simulink model "motorPos_ControlModel"  (R2020a)
settings: Solver=VariableStepAuto  StartTime=0.0  StopTime=10.0  RelTol=1e-3
values from neighbouring files (symbols this model uses):
  Kd = 0.084    [motor_parameter.sldd]
  Ki = 62.72    [motor_parameter.sldd]
  Kp = 4.023    [motor_parameter.sldd]
settings Model: DataDictionary=motor_parameter.sldd  Creator=INDRAJIT MARATHE  LastModifiedBy=INDRAJIT MARATHE

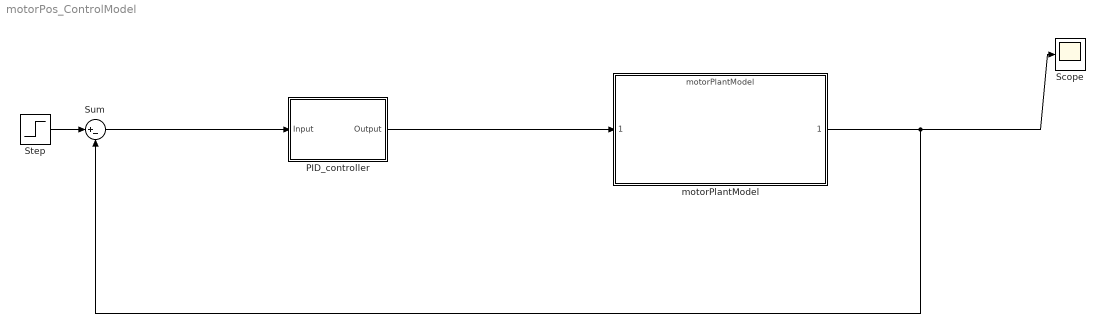
== system motorPos_ControlModel ==
  PID_controller : Subsystem
  Scope : Scope
  Step : Step  SampleTime=0
  Sum : Sum  Inputs=|+-
  motorPlantModel : ModelReference  ModelNameDialog=motorPlantModel  ModelReferenceVersion=1.11
  wires:
  Step/1 -> Sum/1
  motorPlantModel/1 -> Scope/1, Sum/2
  PID_controller/1(Output) -> motorPlantModel/1
  Sum/1 -> PID_controller/1(Input)

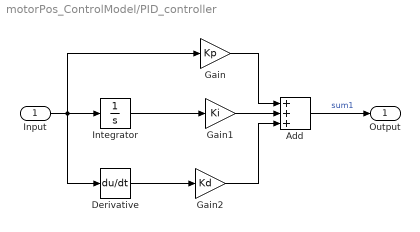
== system motorPos_ControlModel/PID_controller ==
  Input : Inport
  Add : Sum  Inputs=+++
  Derivative : Derivative
  Gain : Gain  Gain=Kp
  Gain1 : Gain  Gain=Ki
  Gain2 : Gain  Gain=Kd
  Integrator : Integrator
  Output : Outport
  wires:
  Add/1 -> Output/1  "sum1"
  Gain/1 -> Add/1
  Integrator/1 -> Gain1/1
  Gain1/1 -> Add/2
  Derivative/1 -> Gain2/1
  Input/1 -> Derivative/1, Integrator/1, Gain/1
  Gain2/1 -> Add/3
